simulink model "H2DFRL_LExCI_env_PPO"  (R2023a)
settings: Solver=FixedStepAuto  StartTime=0.0  StopTime=50  FixedStep=0.08  RelTol=1e-3
values from neighbouring files (symbols this model uses):
  action_mean_selector_ppo = 1:num_actions    [ReinforcementLearningBlockInit_H2DFRL.m]
  action_sampling_mode = 1    [ReinforcementLearningBlockInit_H2DFRL.m]
  action_selector_ddpg = 1:num_actions    [ReinforcementLearningBlockInit_H2DFRL.m]
  action_std_selector_ppo = 1:num_actions    [ReinforcementLearningBlockInit_H2DFRL.m]
  action_type = 1    [ReinforcementLearningBlockInit_H2DFRL.m]
  C2C_NMPC = init_C2C_NMPC_H2DF(C2C_NMPC.expdata)    [init_H2DFRL_GRU.m]
  LowerLimit = ([0.17e-3;350;-5;1e-3] - C2C_NMPC.Normalization.controls.mean)./(C2C_NMPC.Normalization.controls.std)    [init_H2DFRL_GRU.m]
  num_actions = 4    [ReinforcementLearningBlockInit_H2DFRL.m]
  rl_algorithm = 1    [ReinforcementLearningBlockInit_H2DFRL.m]
  UpperLimit = ([0.5e-3;900;2;5.5e-3] - C2C_NMPC.Normalization.controls.mean)./(C2C_NMPC.Normalization.controls.std)    [init_H2DFRL_GRU.m]
undefined symbols (not defined in the file or in its folder): CA50_offset, DiscIntNeverNeededParam, enable_CA50_noise, enable_CA50_offset, enable_IMEP_noise, enable_IMEP_offset, IMEP_offset, NUMBER_OF_ACTIONS
libraries: simulink x23, dspsrcs4 x4
(part 2 of 4)

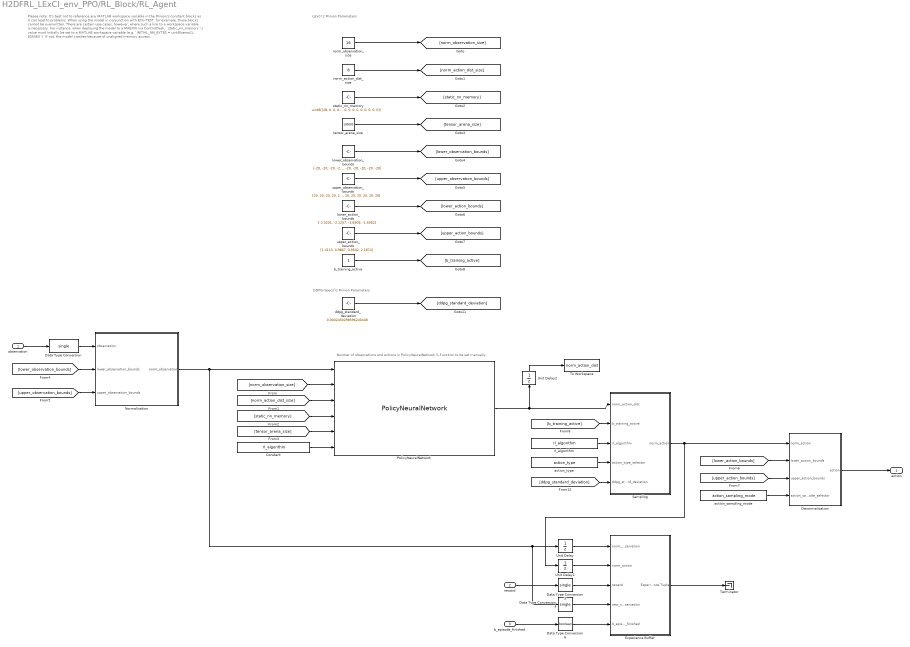
== system H2DFRL_LExCI_env_PPO/RL_Block/RL_Agent ==
  note: LExCI 2 Minion Parameters
  note: DDPG-Specific Minion Parameters
  note: Number of observations and actions in PolicyNeuralNetwork S-Function to be set manually.
  note: Please note:
      |
      | It's best not to reference any MATLAB workspace variable in the Minion's constant blocks as it can lead to
      | problems. When using the model in conjunction with ECU-TEST, for example, those blocks cannot be
      | overwritten.
      |
      | There are certain use-cases, however, where such a link to a workspace variable is necessary. For
      | instance, when deploying the model to a MABXIII via ControlDesk, `static_nn_memory`'s value must
      | initially be set to a MATLAB workspace variable (e.g. `INITIAL_NN_BYTES = uint8(zeros(1, 65536))`). If
      | not, the model crashes because of unaligned memory access.
  observation : Inport
  reward : Inport  Port=2
  b_episode_finished : Inport  Port=3
  Constant : Constant  Value=rl_algorithm  OutDataTypeStr=uint32
  Data Type Conversion : DataTypeConversion  OutDataTypeStr=single  SaturateOnIntegerOverflow=off  RndMeth=Floor
  Data Type Conversion3 : DataTypeConversion  OutDataTypeStr=single  SaturateOnIntegerOverflow=off  RndMeth=Floor
  Data Type Conversion4 : DataTypeConversion  OutDataTypeStr=single  SaturateOnIntegerOverflow=off  RndMeth=Floor
  Data Type Conversion6 : DataTypeConversion  OutDataTypeStr=boolean  SaturateOnIntegerOverflow=off  RndMeth=Floor
  Denormalization : Subsystem
  Experience Buffer : Subsystem
  Normalization : Subsystem
  PolicyNeuralNetwork : S-Function  InitFcn=try, set_param(gcb,'FunctionName','PolicyNeuralNetwork'), end  FunctionName=PolicyNeuralNetwork  SFunctionModules=PolicyNeuralNetwork_wrapper.cpp activations activations_common add add_common add_n arg_min_max assign_variable batch_to_space_nd broadcast_args broadcast_to call_once cast ceil circular_buffer circular_buffer_common comparisons concatenation conv conv_common cumsum depth_to_space depthwise_conv depthwise_conv_common dequantize dequantize_common detection_postprocess div elementwise elu ethosu exp expand_dims fill floor floor_div floor_mod fully_connected fully_connected_common gather gather_nd hard_swish hard_swish_common if kernel_runner kernel_util_micro l2norm l2_pool_2d leaky_relu leaky_relu_common logical logical_common logistic logistic_common log_softmax lstm_eval maximum_minimum micro_tensor_utils mirror_pad mul mul_common neg pack pad pooling pooling_common prelu prelu_common quantize quantize_common read_variable reduce reduce_common reshape resize_bilinear resize_nearest_neighbor round shape slice softmax softmax_common space_to_batch_nd space_to_depth split split_v squared_difference squeeze strided_slice sub sub_common svdf svdf_common tanh transpose transpose_conv unidirectional_sequence_lstm unpack var_handle while zeros_like flatbuffer_conversions op_resolver tensor_utils error_reporter schema_utils kernel_util portable_tensor_utils quantization_util common memory_helpers all_ops_resolver micro_graph micro_error_reporter micro_context micro_profiler test_helpers recording_micro_allocator micro_interpreter micro_time micro_resource_variable test_helper_custom_ops flatbuffer_utils mock_micro_graph debug_log micro_allocation_info system_setup micro_allocator micro_string micro_utils fake_micro_context persistent_arena_buffer_allocator recording_single_arena_buffer_allocator non_persistent_arena_buffer_allocator single_arena_buffer_allocator greedy_memory_planner linear_memory_planner non_persistent_buffer_planner_shim  SFunctionDeploymentMode=off  EnableBusSupport=off  mask(S-Function Builder){}
      mask help: Simulink:masks:SFunctionBuilder_MD
      mask init:
      | val = [[.9  0.75 0.75 1 1 .9 .9 1]',[1 1 0.75 0.75 .9 .9 1 .9]'];try , sys = get_param(gcb,'SfunBuilderFcnName');if isempty(sys), sys = get_param(gcb,'FunctionName'); end,catch, sys = get_param(gcb,'FunctionName'); end
      settings: CopyFcn=set_param(gcbh,'LinkStatus','none')  PreSaveFcn=try, set_param(gcb,'FunctionName','PolicyNeuralNetwork'), end  OpenFcn=sfunctionwizard(gcbh)
      mask Display:
      | plot(val(:,1),val(:,2))
      | disp(sys)
      | port_label('input',1,'norm_observation')
      | port_label('input',2,'norm_observation_size')
      | port_label('input',3,'norm_action_dist_size')
      | port_label('input',4,'static_nn_memory')
      | port_label('input',5,'tensor_arena_size')
      | port_label('input',6,'rl_algorithm')
      | port_label('output',1,'norm_action_dist')
  Sampling : Subsystem
  Terminator : Terminator
  To Workspace : ToWorkspace  VariableName=norm_action_dist  SampleTime=-1
  Unit Delay : UnitDelay  InitialCondition=-1*ones(16,1)  SampleTime=-1  HasFrameUpgradeWarning=on
  Unit Delay1 : UnitDelay  InitialCondition=-1*ones(4,1)  SampleTime=-1  HasFrameUpgradeWarning=on
  Unit Delay2 : UnitDelay  InitialCondition=-1*ones(8,1)  SampleTime=-1  HasFrameUpgradeWarning=on
  action_sampling_mode : Constant  Value=action_sampling_mode  OutDataTypeStr=uint8
  action_type : Constant  Value=action_type  OutDataTypeStr=uint8
  b_training_active : Constant  OutDataTypeStr=boolean
  ddpg_standard_deviation : Constant  Value=0.0002450298596240448  OutDataTypeStr=single
  lower_action_bounds : Constant  Value=[-2.3201, -2.1257, -1.8309, -1.6562]  OutDataTypeStr=single
  lower_observation_bounds : Constant  Value=[-20, -20, -20, -20, -20, -20, -20, -20, -20, -20, -20, -20, -20, -20, -20, -20]  OutDataTypeStr=single
  norm_action_dist_size : Constant  Value=8  OutDataTypeStr=uint32
  norm_observation_size : Constant  Value=16  OutDataTypeStr=uint32
  rl_algorithm : Constant  Value=rl_algorithm  OutDataTypeStr=uint8
  static_nn_memory : Constant  Value=uint8([28, 0, 0, 0, 84, 70, 76, 51, 0, 0, 18, 0, 28, 0, 24, 0, 20, 0, 16, 0, 12, 0, 8, 0, 0, 0, 4, 0, 18, 0, 0, 0, 24, 0, 0, 0, 104, 0, 0, 0, 88, 30, 0, 0, 104, 30, 0, 0, 176, 42, 0, 0, 3, 0, 0, 0, 2, 0, 0, 0, 44, 0, 0, 0, 4, 0, 0, 0, 204, 221, 255, 255, 33, 0, 0, 0, 4, 0, 0, 0, 19, 0, 0, 0, 67, 79, 78, 86, 69, 82, 83, 73, 79, 78, 95, 77, 69, 84, 65, 68, 65, 84, 65, 0, 240, 221, 255, 255, 32, 0, 0, 0, 4, 0, 0, 0, 19, 0, 0, 0, 109, 105, 110, 95, 114, 117, 110, 116, 105, 109, 101, 95, 118, 101, 114, 115, 105, 111, 110, 0, 34, 0, 0, 0, 236, 29, 0, 0, 220, 27, 0, 0, 132, 27, 0, 0, 116, 23, 0, 0, 100, 19, 0, 0, 84, 15, 0, 0, 4, 15, 0, 0, 244, 10, 0, 0, 164, 10, 0, 0, 148, 6, 0, 0, 140, 6, 0, 0, 120, 6, 0, 0, 104, 2, 0, 0, 56, 2, 0, 0, 48, 2, 0, 0, 224, 1, 0, 0, 216, 1, 0, 0, 136, 1, 0, 0, 128, 1, 0, 0, 120, 1, 0, 0, 40, 1, 0, 0, 32, 1, 0, 0, 24, 1, 0, 0, 16, 1, 0, 0, 192, 0, 0, 0, 184, 0, 0, 0, 176, 0, 0, 0, 168, 0, 0, 0, 160, 0, 0, 0, 152, 0, 0, 0, 144, 0, 0, 0, 136, 0, 0, 0, 104, 0, 0, 0, 4, 0, 0, 0, 174, 228, 255, 255, 4, 0, 0, 0, 84, 0, 0, 0, 12, 0, 0, 0, 8, 0, 14, 0, 8, 0, 4, 0, 8, 0, 0, 0, 16, 0, 0, 0, 36, 0, 0, 0, 0, 0, 6, 0, 8, 0, 4, 0, 6, 0, 0, 0, 4, 0, 0, 0, 0, 0, 0, 0, 0, 0, 10, 0, 16, 0, 12, 0, 8, 0, 4, 0, 10, 0, 0, 0, 2, 0, 0, 0, 2, 0, 0, 0, 4, 0, 0, 0, 6, 0, 0, 0, 50, 46, 49, 49, 46, 48, 0, 0, 14, 229, 255, 255, 4, 0, 0, 0, 16, 0, 0, 0, 49, 46, 49, 52, 46, 48, 0, 0, 0, 0, 0, 0, 0, 0, 0, 0, 216, 214, 255, 255, 220, 214, 255, 255, 224, 214, 255, 255, 228, 214, 255, 255, 232, 214, 255, 255, 236, 214, 255, 255, 240, 214, 255, 255, 70, 229, 255, 255, 4, 0, 0, 0, 64, 0, 0, 0, 182, 224, 143, 188, 131, 172, 76, 60, 11, 225, 49, 189, 9, 183, 231, 188, 58, 185, 172, 188, 72, 115, 139, 188, 78, 66, 3, 189, 26, 88, 40, 189, 215, 203, 2, 189, 28, 91, 226, 189, 48, 116, 79, 61, 194, 231, 68, 61, 185, 103, 218, 189, 62, 14, 204, 61, 215, 215, 122, 62, 182, 14, 226, 61, 64, 215, 255, 255, 68, 215, 255, 255, 72, 215, 255, 255, 158, 229, 255, 255, 4, 0, 0, 0, 64, 0, 0, 0, 95, 59, 164, 62, 182, 22, 135, 190, 90, 71, 128, 190, 7, 84, 181, 190, 195, 65, 123, 190, 186, 147, 126, 62, 61, 95, 140, 190, 105, 179, 122, 62, 147, 66, 127, 190, 230, 93, 157, 62, 188, 75, 144, 62, 73, 71, 125, 190, 60, 248, 166, 190, 73, 191, 160, 190, 201, 151, 123, 62, 183, 76, 137, 62, 152, 215, 255, 255, 156, 215, 255, 255, 242, 229, 255, 255, 4, 0, 0, 0, 64, 0, 0, 0, 241, 52, 87, 61, 224, 71, 238, 188, 58, 225, 128, 61, 78, 0, 7, 190, 206, 130, 30, 62, 167, 45, 169, 61, 184, 33, 209, 189, 104, 185, 178, 189, 118, 86, 42, 61, 99, 208, 130, 189, 226, 144, 86, 188, 57, 154, 147, 189, 209, 221, 22, 62, 166, 8, 33, 188, 50, 225, 16, 62, 28, 129, 14, 189, 236, 215, 255, 255, 66, 230, 255, 255, 4, 0, 0, 0, 64, 0, 0, 0, 65, 69, 63, 187, 39, 65, 53, 62, 90, 233, 44, 62, 57, 11, 145, 188, 185, 102, 21, 62, 222, 202, 134, 189, 76, 221, 71, 62, 227, 48, 49, 190, 203, 243, 10, 62, 255, 25, 41, 61, 52, 130, 88, 61, 196, 64, 40, 62, 121, 216, 57, 189, 33, 155, 83, 189, 240, 253, 68, 189, 61, 172, 21, 190, 60, 216, 255, 255, 146, 230, 255, 255, 4, 0, 0, 0, 32, 0, 0, 0, 133, 135, 9, 189, 206, 114, 3, 189, 160, 7, 9, 189, 180, 124, 2, 189, 227, 171, 49, 190, 72, 110, 50, 190, 177, 58, 48, 190, 149, 97, 52, 190, 190, 230, 255, 255, 4, 0, 0, 0, 0, 4, 0, 0, 200, 255, 160, 61, 163, 50, 248, 62, 181, 187, 187, 190, 149, 99, 10, 62, 194, 84, 217, 190, 222, 111, 218, 190, 150, 92, 250, 62, 3, 104, 225, 60, 204, 81, 13, 191, 109, 242, 165, 62, 171, 146, 218, 60, 163, 126, 221, 61, 51, 128, 244, 190, 131, 17, 22, 189, 67, 6, 165, 190, 174, 204, 3, 63, 219, 230, 62, 190, 217, 54, 74, 190, 235, 52, 32, 191, 192, 73, 105, 61, 192, 138, 125, 189, 202, 86, 132, 60, 52, 236, 161, 189, 126, 143, 143, 190, 140, 138, 182, 61, 130, 2, 216, 189, 237, 183, 255, 62, 176, 189, 197, 60, 185, 124, 133, 190, 41, 14, 55, 63, 219, 247, 61, 191, 240, 107, 59, 61, 143, 142, 248, 62, 172, 49, 224, 190, 43, 108, 151, 62, 47, 215, 82, 190, 248, 238, 89, 62, 217, 240, 226, 60, 196, 109, 189, 190, 66, 176, 31, 62, ...(+206334 chars)])  OutDataTypeStr=uint8
  tensor_arena_size : Constant  Value=100000  OutDataTypeStr=uint32
  upper_action_bounds : Constant  Value=[1.4113, 0.9867, 0.9542, 2.1874]  OutDataTypeStr=single
  upper_observation_bounds : Constant  Value=[20, 20, 20, 20, 20, 20, 20, 20, 20, 20, 20, 20, 20, 20, 20, 20]  OutDataTypeStr=single
  action : Outport
  wires:
  upper_action_bounds/1 -> [upper_action_bounds]
  PolicyNeuralNetwork/1 -> Unit Delay2/1, Sampling/1(norm_action_dist)
  upper_observation_bounds/1 -> [upper_observation_bounds]
  lower_action_bounds/1 -> [lower_action_bounds]
  [upper_observation_bounds] -> Normalization/3(upper_observation_bounds)
  [tensor_arena_size] -> PolicyNeuralNetwork/5
  b_episode_finished/1 -> Data Type Conversion6/1
  Unit Delay/1 -> Experience Buffer/1(norm_observation)
  [norm_observation_size] -> PolicyNeuralNetwork/2
  Data Type Conversion6/1 -> Experience Buffer/5(b_episode_finished)
  Unit Delay1/1 -> Experience Buffer/2(norm_action)
  Data Type Conversion3/1 -> Experience Buffer/3(reward)
  norm_observation_size/1 -> [norm_observation_size]
  Data Type Conversion/1 -> Normalization/1(observation)
  lower_observation_bounds/1 -> [lower_observation_bounds]
  Data Type Conversion4/1 -> Experience Buffer/4(new_norm_observation)
  reward/1 -> Data Type Conversion3/1
  norm_action_dist_size/1 -> [norm_action_dist_size]
  static_nn_memory/1 -> [static_nn_memory]
  Normalization/1(norm_observation) -> Unit Delay/1, Data Type Conversion4/1, PolicyNeuralNetwork/1
  observation/1 -> Data Type Conversion/1
  [norm_action_dist_size] -> PolicyNeuralNetwork/3
  [lower_observation_bounds] -> Normalization/2(lower_observation_bounds)
  tensor_arena_size/1 -> [tensor_arena_size]
  Experience Buffer/1(Experience Tuple) -> Terminator/1
  Sampling/1(norm_action) -> Unit Delay1/1, Denormalization/1(norm_action)
  Denormalization/1(action) -> action/1
  [lower_action_bounds] -> Denormalization/2(lower_action_bounds)
  [upper_action_bounds] -> Denormalization/3(upper_action_bounds)
  [static_nn_memory] -> PolicyNeuralNetwork/4
  b_training_active/1 -> [b_training_active]
  [b_training_active] -> Sampling/2(b_training_active)
  ddpg_standard_deviation/1 -> [ddpg_standard_deviation]
  action_sampling_mode/1 -> Denormalization/4(action_sampling_mode_selector)
  action_type/1 -> Sampling/4(action_type_selector)
  rl_algorithm/1 -> Sampling/3(rl_algorithm)
  [ddpg_standard_deviation] -> Sampling/5(ddpg_standard_deviation)
  Constant/1 -> PolicyNeuralNetwork/6
  Unit Delay2/1 -> To Workspace/1
